simulink model "Teleoperation_no_voltage"  (R2020a)
settings: Solver=VariableStepAuto  StartTime=0.0  StopTime=7  RelTol=1e-3
values from neighbouring files (symbols this model uses):
  B = 1 / k_m    (= 0.0517063081696)    [Teleop_parameters.m]    (also in base.mat; base_no_attrito.mat = 0; ci_siamo.mat; force_control.mat)
  Be = 5    [Teleop_parameters.m]    (also in base.mat = 0.5; base_no_attrito.mat = 0.5; ci_siamo.mat; force_control.mat = 0.5)
  Bh = 0.02    [Teleop_parameters.m]    (also in base.mat; base_no_attrito.mat; ci_siamo.mat; force_control.mat)
  Fc_h = 5    [Teleop_parameters.m]    (also in base.mat; base_no_attrito.mat; ci_siamo.mat; force_control.mat)
  J = tau_m / k_m    (= 0.0629265770424)    [Teleop_parameters.m]    (also in base.mat; base_no_attrito.mat; ci_siamo.mat; force_control.mat)
  J_r = 1e-1    (= 0.1)    [Teleop_parameters.m]    (also in base.mat = 0.0943898655636; base_no_attrito.mat = 0.0943898655636; ci_siamo.mat = 0.0629265770424; force_control.mat = 0.0943898655636)
  Jh = 0.02    [Teleop_parameters.m]    (also in base.mat; base_no_attrito.mat; ci_siamo.mat; force_control.mat)
  Kc2v_m = 2    [Teleop_parameters.m]    (also in base.mat; base_no_attrito.mat; ci_siamo.mat; force_control.mat)
  Kc2v_s = 2    [Teleop_parameters.m]    (also in base.mat; base_no_attrito.mat; ci_siamo.mat; force_control.mat)
  Kd_h = 10    [Teleop_parameters.m]    (also in base.mat = 1; base_no_attrito.mat = 1; ci_siamo.mat; force_control.mat = 1)
  Kd_m = 0.005    [Teleop_parameters.m]    (also in base.mat = 1; base_no_attrito.mat = 1; ci_siamo.mat; force_control.mat = 1)
  Kd_s = 0.5    [Teleop_parameters.m]    (also in base.mat = 1; base_no_attrito.mat = 1; ci_siamo.mat; force_control.mat = 1)
  Ke = 1000    [Teleop_parameters.m]    (also in base.mat = 10; base_no_attrito.mat = 10; ci_siamo.mat = 10; force_control.mat = 10)
  Kp_h = 10    [Teleop_parameters.m]    (also in base.mat = 1.2; base_no_attrito.mat = 1.2; ci_siamo.mat; force_control.mat = 1.2)
  Kp_m = 0.01    [Teleop_parameters.m]    (also in base.mat = 1; base_no_attrito.mat = 1; ci_siamo.mat; force_control.mat = 1)
  Kp_s = 1    [Teleop_parameters.m]    (also in base.mat; base_no_attrito.mat; ci_siamo.mat; force_control.mat)
  Kt2c_m = 1.182    [Teleop_parameters.m]    (also in base.mat; base_no_attrito.mat; ci_siamo.mat; force_control.mat)
  Kt2c_s = 1.182    [Teleop_parameters.m]    (also in base.mat; base_no_attrito.mat; ci_siamo.mat; force_control.mat)
  Kv_fc = 10    [Teleop_parameters.m]    (also in base.mat = 0; base_no_attrito.mat = 0; ci_siamo.mat; force_control.mat = 30)
  lArm_m = 0.1    [Teleop_parameters.m]    (also in base.mat; base_no_attrito.mat; ci_siamo.mat; force_control.mat)
  lArm_s = 0.1    [Teleop_parameters.m]    (also in base.mat; base_no_attrito.mat; ci_siamo.mat; force_control.mat)
  qe = 0.5    [Teleop_parameters.m]    (also in base.mat = 5; base_no_attrito.mat = 5; ci_siamo.mat; force_control.mat = 5)
settings Model: Creator=gbagolin  LastModifiedBy=giova

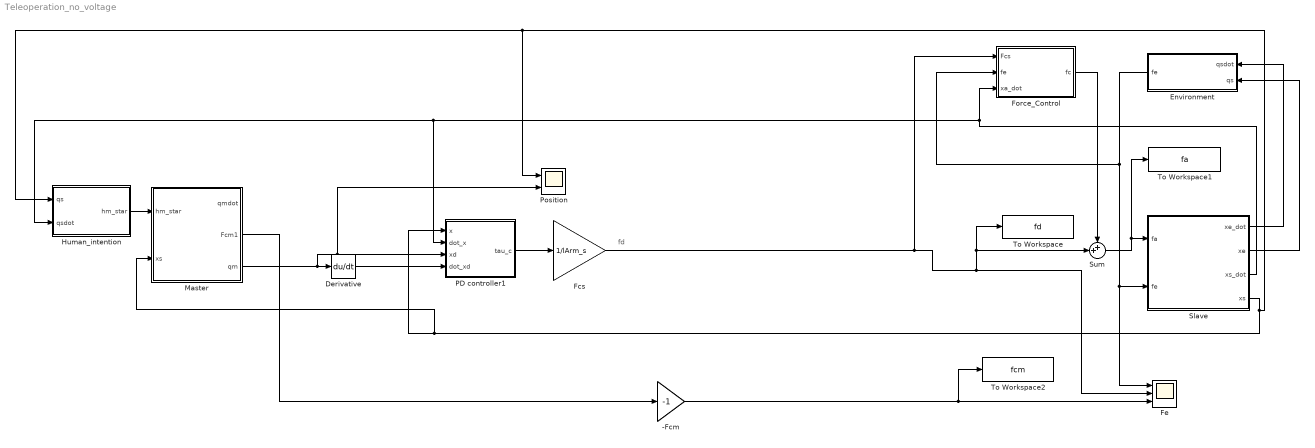
== system Teleoperation_no_voltage ==
  note: fd
  -Fcm : Gain  Gain=-1
  Derivative : Derivative
  Environment : Subsystem
  Fcs : Gain  Gain=1/lArm_s
  Fe : Scope  NumInputPorts=3
  Force_Control : Subsystem
  Human_intention : Subsystem
  Master : Subsystem
  PD controller1 : Subsystem
  Position : Scope  NumInputPorts=2
  Slave : Subsystem
  Sum : Sum  Inputs=++|
  To Workspace : ToWorkspace  VariableName=fd  SaveFormat=Timeseries  SampleTime=-1
  To Workspace1 : ToWorkspace  VariableName=fa  SaveFormat=Timeseries  SampleTime=-1
  To Workspace2 : ToWorkspace  VariableName=fcm  SaveFormat=Timeseries  SampleTime=-1
  wires:
  Human_intention/1(hm_star) -> Master/1(hm_star)
  Fcs/1 -> Sum/2, To Workspace/1, Fe/2, Force_Control/1(Fcs)
  Sum/1 -> To Workspace1/1, Slave/1(fa)
  Environment/1(fe) -> Force_Control/2(fe), Fe/1, Slave/2(fe)
  -Fcm/1 -> Fe/3, To Workspace2/1
  Force_Control/1(fc) -> Sum/1
  Slave/3(xs_dot) -> Force_Control/3(xa_dot), Human_intention/2(qsdot), PD controller1/2(dot_x)
  Slave/1(xe_dot) -> Environment/1(qsdot)
  Slave/2(xe) -> Environment/2(qs)
  Slave/4(xs) -> Master/2(xs), PD controller1/1(x), Position/1, Human_intention/1(qs)
  Master/2(Fcm1) -> -Fcm/1
  PD controller1/1(tau_c) -> Fcs/1
  Master/3(qm) -> Derivative/1, Position/2, PD controller1/3(xd)
  Derivative/1 -> PD controller1/4(dot_xd)

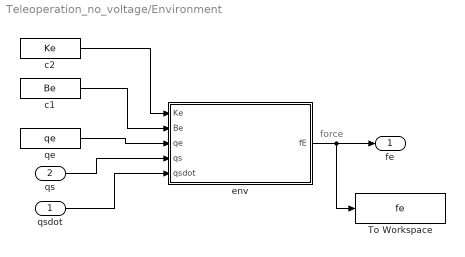
== system Teleoperation_no_voltage/Environment ==
  note: force
  qsdot : Inport
  qs : Inport  Port=2
  To Workspace : ToWorkspace  VariableName=fe  SaveFormat=Timeseries  SampleTime=-1
  c1 : Constant  Value=Be  SampleTime=0
  c2 : Constant  Value=Ke  SampleTime=0
  env : MATLAB Function  TreatAsAtomicUnit=on
  qe : Constant  Value=qe  SampleTime=0
  fe : Outport  VectorParamsAs1DForOutWhenUnconnected=off
  wires:
  qe/1 -> env/3(qe)
  c1/1 -> env/2(Be)
  c2/1 -> env/1(Ke)
  qs/1 -> env/4(qs)
  qsdot/1 -> env/5(qsdot)
  env/1(fE) -> To Workspace/1, fe/1

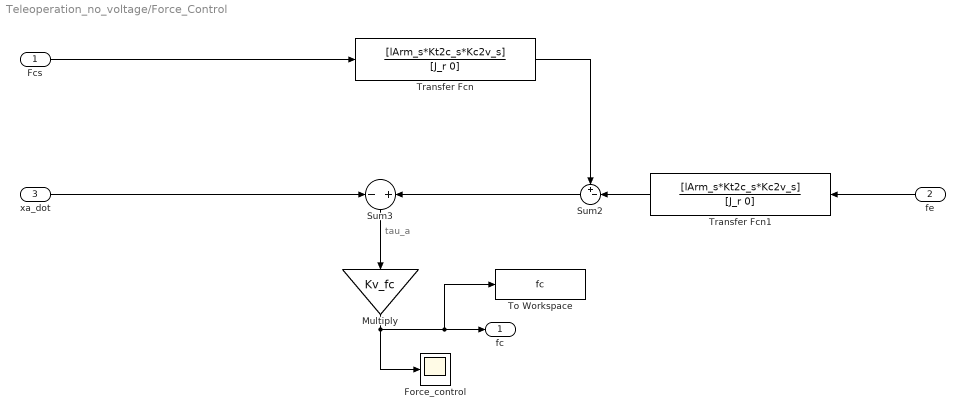
== system Teleoperation_no_voltage/Force_Control ==
  note: tau_a
  Fcs : Inport
  fe : Inport  Port=2
  xa_dot : Inport  Port=3
  Force_control : Scope
  Multiply : Gain  Gain=Kv_fc
  Sum2 : Sum  Inputs=+-|
  Sum3 : Sum  Inputs=-|+
  To Workspace : ToWorkspace  VariableName=fc  SaveFormat=Timeseries  SampleTime=-1
  Transfer Fcn : TransferFcn  Numerator=[lArm_s*Kt2c_s*Kc2v_s]  Denominator=[J_r 0]
  Transfer Fcn1 : TransferFcn  Numerator=[lArm_s*Kt2c_s*Kc2v_s]  Denominator=[J_r 0]
  fc : Outport
  wires:
  Transfer Fcn1/1 -> Sum2/2
  Sum2/1 -> Sum3/2
  Sum3/1 -> Multiply/1
  Multiply/1 -> To Workspace/1, fc/1, Force_control/1
  Fcs/1 -> Transfer Fcn/1
  fe/1 -> Transfer Fcn1/1
  xa_dot/1 -> Sum3/1
  Transfer Fcn/1 -> Sum2/1

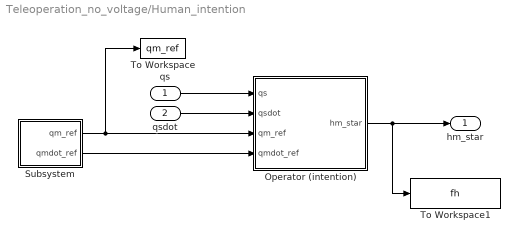
== system Teleoperation_no_voltage/Human_intention ==
  qs : Inport
  qsdot : Inport  Port=2
  Operator (intention) : Subsystem
  Subsystem : Subsystem
  To Workspace : ToWorkspace  VariableName=qm_ref  SaveFormat=Timeseries  SampleTime=-1
  To Workspace1 : ToWorkspace  VariableName=fh  SaveFormat=Timeseries  SampleTime=-1
  hm_star : Outport
  wires:
  Subsystem/1(qm_ref) -> To Workspace/1, Operator (intention)/3(qm_ref)
  Subsystem/2(qmdot_ref) -> Operator (intention)/4(qmdot_ref)
  Operator (intention)/1(hm_star) -> To Workspace1/1, hm_star/1
  qs/1 -> Operator (intention)/1(qs)
  qsdot/1 -> Operator (intention)/2(qsdot)

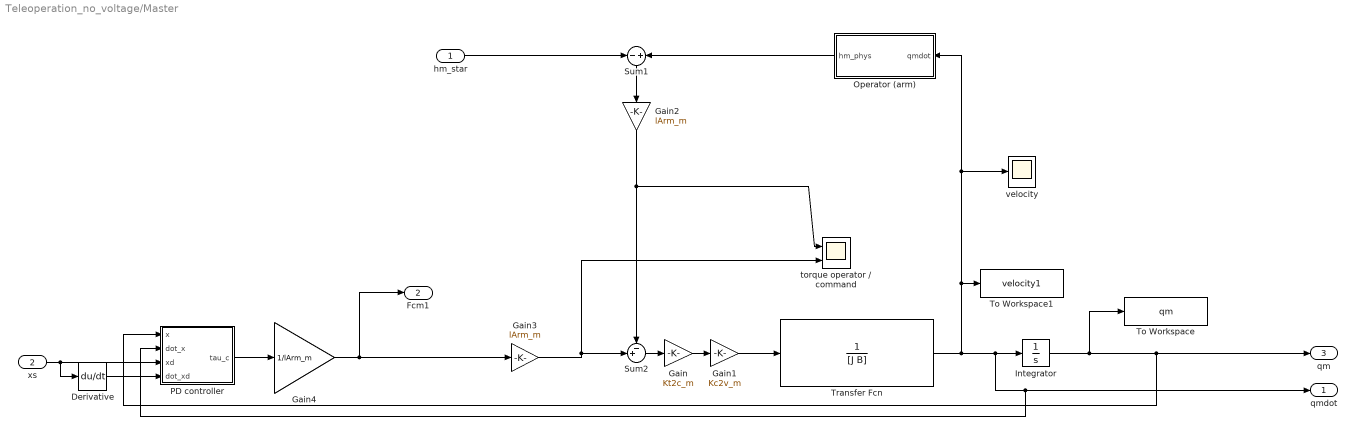
== system Teleoperation_no_voltage/Master ==
  hm_star : Inport
  xs : Inport  Port=2
  Derivative : Derivative
  Gain : Gain  Gain=Kt2c_m
  Gain1 : Gain  Gain=Kc2v_m
  Gain2 : Gain  Gain=lArm_m
  Gain3 : Gain  Gain=lArm_m
  Gain4 : Gain  Gain=1/lArm_m
  Integrator : Integrator
  Operator (arm) : Subsystem
  PD controller : Subsystem
  Sum1 : Sum  Inputs=-+
  Sum2 : Sum  Inputs=-+|
  To Workspace : ToWorkspace  VariableName=qm  SaveFormat=Timeseries  SampleTime=-1
  To Workspace1 : ToWorkspace  VariableName=velocity1  SaveFormat=Timeseries  SampleTime=-1
  Transfer Fcn : TransferFcn  Denominator=[J B]
  torque operator / command : Scope  NumInputPorts=2
  velocity : Scope
  qmdot : Outport
  Fcm1 : Outport  Port=2
  qm : Outport  Port=3
  wires:
  Integrator/1 -> To Workspace/1, PD controller/1(x), qm/1
  Operator (arm)/1(hm_phys) -> Sum1/2
  Sum1/1 -> Gain2/1
  Gain4/1 -> Fcm1/1, Gain3/1
  Transfer Fcn/1 -> Operator (arm)/1(qmdot), velocity/1, To Workspace1/1, PD controller/2(dot_x), qmdot/1, Integrator/1
  hm_star/1 -> Sum1/1
  Sum2/1 -> Gain/1
  Gain/1 -> Gain1/1
  Gain1/1 -> Transfer Fcn/1
  Gain2/1 -> Sum2/1, torque operator / command/1
  Gain3/1 -> torque operator / command/2, Sum2/2
  Derivative/1 -> PD controller/4(dot_xd)
  xs/1 -> Derivative/1, PD controller/3(xd)
  PD controller/1(tau_c) -> Gain4/1

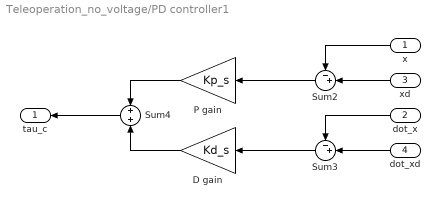
== system Teleoperation_no_voltage/PD controller1 ==
  x : Inport
  dot_x : Inport  Port=2
  xd : Inport  Port=3
  dot_xd : Inport  Port=4
  D gain : Gain  Gain=Kd_s
  P gain : Gain  Gain=Kp_s
  Sum2 : Sum  Inputs=-+|
  Sum3 : Sum  Inputs=-+|
  Sum4 : Sum
  tau_c : Outport  VectorParamsAs1DForOutWhenUnconnected=off
  wires:
  D gain/1 -> Sum4/2
  dot_x/1 -> Sum3/1
  dot_xd/1 -> Sum3/2
  x/1 -> Sum2/1
  xd/1 -> Sum2/2
  Sum3/1 -> D gain/1
  P gain/1 -> Sum4/1
  Sum4/1 -> tau_c/1
  Sum2/1 -> P gain/1

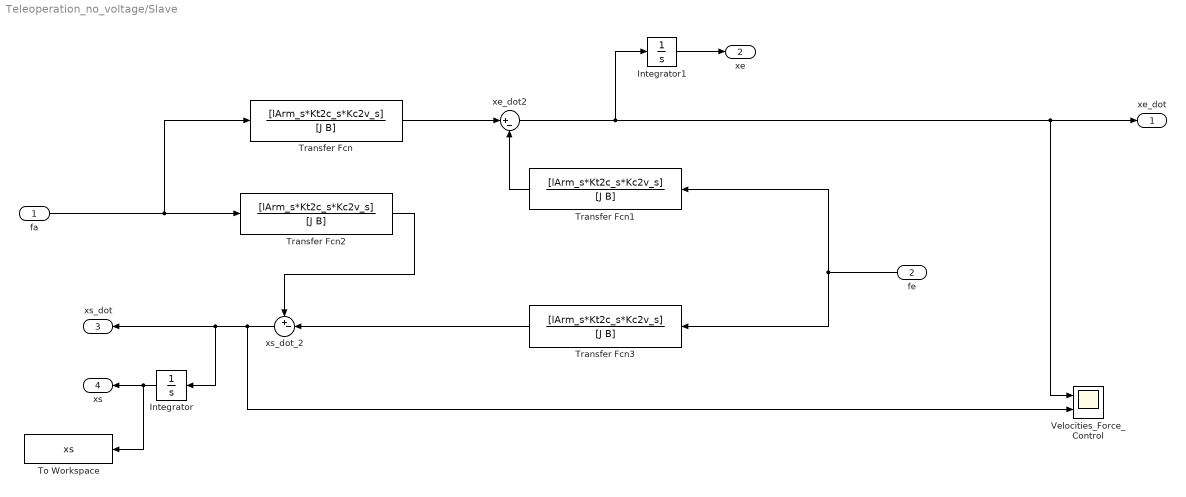
== system Teleoperation_no_voltage/Slave ==
  fa : Inport
  fe : Inport  Port=2
  Integrator : Integrator
  Integrator1 : Integrator
  To Workspace : ToWorkspace  VariableName=xs  SaveFormat=Timeseries  SampleTime=-1
  Transfer Fcn{,1..3} (4 alike) : TransferFcn  Numerator=[lArm_s*Kt2c_s*Kc2v_s]  Denominator=[J B]
  Velocities_Force_Control : Scope  NumInputPorts=2
  xe_dot2 : Sum  Inputs=|+-
  xs_dot_2 : Sum  Inputs=+-|
  xe_dot : Outport
  xe : Outport  Port=2
  xs_dot : Outport  Port=3
  xs : Outport  Port=4
  wires:
  fa/1 -> Transfer Fcn2/1, Transfer Fcn/1
  Transfer Fcn/1 -> xe_dot2/1
  xe_dot2/1 -> Integrator1/1, xe_dot/1, Velocities_Force_Control/1
  Transfer Fcn1/1 -> xe_dot2/2
  Transfer Fcn3/1 -> xs_dot_2/2
  Transfer Fcn2/1 -> xs_dot_2/1
  xs_dot_2/1 -> Velocities_Force_Control/2, Integrator/1, xs_dot/1
  fe/1 -> Transfer Fcn1/1, Transfer Fcn3/1
  Integrator/1 -> To Workspace/1, xs/1
  Integrator1/1 -> xe/1

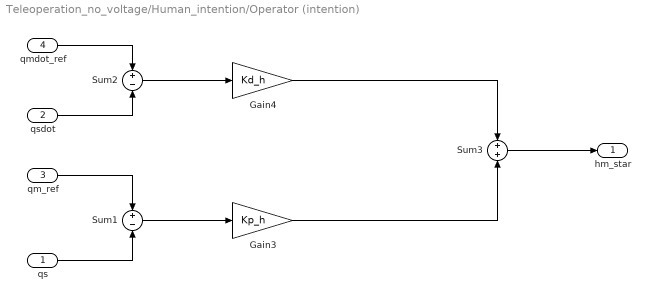
== system Teleoperation_no_voltage/Human_intention/Operator (intention) ==
  qs : Inport
  qsdot : Inport  Port=2
  qm_ref : Inport  Port=3
  qmdot_ref : Inport  Port=4
  Gain3 : Gain  Gain=Kp_h
  Gain4 : Gain  Gain=Kd_h
  Sum1 : Sum  Inputs=+|-
  Sum2 : Sum  Inputs=+|-
  Sum3 : Sum  Inputs=+|+
  hm_star : Outport  VectorParamsAs1DForOutWhenUnconnected=off
  wires:
  qs/1 -> Sum1/2
  qm_ref/1 -> Sum1/1
  qmdot_ref/1 -> Sum2/1
  Sum1/1 -> Gain3/1
  qsdot/1 -> Sum2/2
  Sum2/1 -> Gain4/1
  Gain4/1 -> Sum3/1
  Gain3/1 -> Sum3/2
  Sum3/1 -> hm_star/1

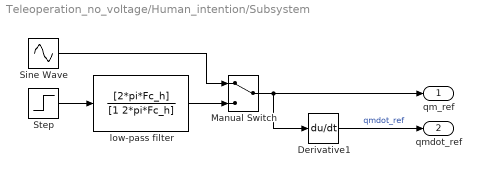
== system Teleoperation_no_voltage/Human_intention/Subsystem ==
  Derivative1 : Derivative  CoefficientInTFapproximation=0.001
  Manual Switch : ManualSwitch
  Sine Wave : Sin  SampleTime=0
  Step : Step  SampleTime=0
  low-pass filter : TransferFcn  Numerator=[2*pi*Fc_h]  Denominator=[1 2*pi*Fc_h]
  qm_ref : Outport
  qmdot_ref : Outport  Port=2
  wires:
  low-pass filter/1 -> Manual Switch/2
  Manual Switch/1 -> qm_ref/1, Derivative1/1
  Derivative1/1 -> qmdot_ref/1  "qmdot_ref"
  Step/1 -> low-pass filter/1
  Sine Wave/1 -> Manual Switch/1

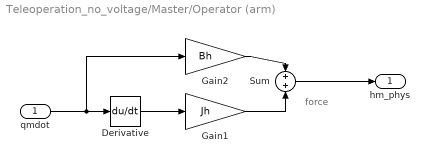
== system Teleoperation_no_voltage/Master/Operator (arm) ==
  note: force
  qmdot : Inport
  Derivative : Derivative  CoefficientInTFapproximation=0.001
  Gain1 : Gain  Gain=Jh
  Gain2 : Gain  Gain=Bh
  Sum : Sum  Inputs=+|+
  hm_phys : Outport  VectorParamsAs1DForOutWhenUnconnected=off
  wires:
  qmdot/1 -> Gain2/1, Derivative/1
  Sum/1 -> hm_phys/1
  Derivative/1 -> Gain1/1
  Gain2/1 -> Sum/1
  Gain1/1 -> Sum/2

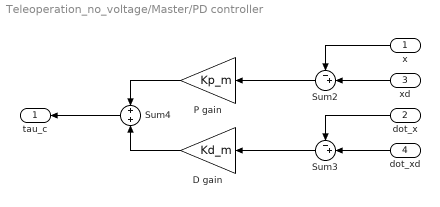
== system Teleoperation_no_voltage/Master/PD controller ==
  x : Inport
  dot_x : Inport  Port=2
  xd : Inport  Port=3
  dot_xd : Inport  Port=4
  D gain : Gain  Gain=Kd_m
  P gain : Gain  Gain=Kp_m
  Sum2 : Sum  Inputs=-+|
  Sum3 : Sum  Inputs=-+|
  Sum4 : Sum
  tau_c : Outport  VectorParamsAs1DForOutWhenUnconnected=off
  wires:
  D gain/1 -> Sum4/2
  dot_x/1 -> Sum3/1
  dot_xd/1 -> Sum3/2
  x/1 -> Sum2/1
  xd/1 -> Sum2/2
  Sum3/1 -> D gain/1
  P gain/1 -> Sum4/1
  Sum4/1 -> tau_c/1
  Sum2/1 -> P gain/1

== matlab function Teleoperation_no_voltage/Environment/env ==
  data: Ke input; Be input; qe input; qs input; fE output; qsdot input
function fE  = environment(Ke, Be, qe, qs, qsdot)
if qs > qe
   fE = Ke * (qs - qe) + Be * qsdot;
else
   fE = 0;
end
